simulink library "halout"  (R2021b)
settings: Solver=VariableStepAuto  StartTime=0.0  StopTime=10.0  RelTol=1e-3
undefined symbols (not defined in the file): C_TASK_5MS_S, FALSE, KHAL_CAN1FD1APS3E2E_flg, KHAL_CAN1FD1APS3TxReq_flg, KHAL_CAN1FD1VCU2E2E_flg, KHAL_CAN1FD1VCU2TxReq_flg, KHAL_CAN1FD1VCU3E2E_flg, KHAL_CAN1FD1VCU3TxReq_flg, KHAL_CAN1TxReq_flg, KHAL_CAN1VMCFCM1E2E_flg, KHAL_CAN1VMCFCM1TxReq_flg, KHAL_CAN2TxReq_flg, KHAL_CAN3FD3VCU1toNIDECTxReq_flg, KHAL_CAN3FD3VCU1TxReq_flg, KHAL_CAN3FD3VCU2E2E_flg, KHAL_CAN3FD3VCU2toNIDECE2E_flg, KHAL_CAN3FD3VCU2toNIDECTxReq_flg, KHAL_CAN3FD3VCU2TxReq_flg, KHAL_CAN3TxReq_flg, KHAL_CAN4FD4CE1000E2E_flg, KHAL_CAN4FD4CE1000TxReq_flg, KHAL_CAN4TxReq_flg, KHAL_CAN5TxReq_flg, KHAL_CAN6FD6APS3E2E_flg, KHAL_CAN6FD6APS3TxReq_flg, KHAL_CAN6FD6VCU2E2E_flg, KHAL_CAN6FD6VCU2TxReq_flg, KHAL_CAN6TxReq_flg, ONE_INT, TRUE, ZERO_INT
libraries: FVT_lib x549, simulink x244
(part 18 of 27)

== system halout/HAL_OUT/CAN2/FD2_CE100_0_0x117/FDCBCMHMIKey2FuncSta ==
  FDCBCMHMIKey2FuncSta : Inport
  Data Type Conversion : DataTypeConversion  OutDataTypeStr=uint8  RndMeth=Round
  CAN2_FDC_BCM_HMIKey2Func_Sta : Outport
  wires:
  Data Type Conversion/1 -> CAN2_FDC_BCM_HMIKey2Func_Sta/1
  FDCBCMHMIKey2FuncSta/1 -> Data Type Conversion/1

== system halout/HAL_OUT/CAN2/FD2_CE100_0_0x117/FDCBCMHMIKey3FuncSta ==
  FDCBCMHMIKey3FuncSta : Inport
  Data Type Conversion : DataTypeConversion  OutDataTypeStr=uint8  RndMeth=Round
  CAN2_FDC_BCM_HMIKey3Func_Sta : Outport
  wires:
  Data Type Conversion/1 -> CAN2_FDC_BCM_HMIKey3Func_Sta/1
  FDCBCMHMIKey3FuncSta/1 -> Data Type Conversion/1

== system halout/HAL_OUT/CAN2/FD2_CE100_0_0x117/FDCBCMHMIKey4FuncSta ==
  FDCBCMHMIKey4FuncSta : Inport
  Data Type Conversion : DataTypeConversion  OutDataTypeStr=uint8  RndMeth=Round
  CAN2_FDC_BCM_HMIKey4Func_Sta : Outport
  wires:
  Data Type Conversion/1 -> CAN2_FDC_BCM_HMIKey4Func_Sta/1
  FDCBCMHMIKey4FuncSta/1 -> Data Type Conversion/1

== system halout/HAL_OUT/CAN2/FD2_CE100_0_0x117/FDCBCMHMIKey5FuncSta ==
  FDCBCMHMIKey5FuncSta : Inport
  Data Type Conversion : DataTypeConversion  OutDataTypeStr=uint8  RndMeth=Round
  CAN2_FDC_BCM_HMIKey5Func_Sta : Outport
  wires:
  Data Type Conversion/1 -> CAN2_FDC_BCM_HMIKey5Func_Sta/1
  FDCBCMHMIKey5FuncSta/1 -> Data Type Conversion/1

== system halout/HAL_OUT/CAN2/FD2_CE100_0_0x117/FDCBCMHMIKey6FuncSta ==
  FDCBCMHMIKey6FuncSta : Inport
  Data Type Conversion : DataTypeConversion  OutDataTypeStr=uint8  RndMeth=Round
  CAN2_FDC_BCM_HMIKey6Func_Sta : Outport
  wires:
  Data Type Conversion/1 -> CAN2_FDC_BCM_HMIKey6Func_Sta/1
  FDCBCMHMIKey6FuncSta/1 -> Data Type Conversion/1

== system halout/HAL_OUT/CAN2/FD2_CE100_0_0x117/FDCBCMHMIKey7FuncSta ==
  FDCBCMHMIKey7FuncSta : Inport
  Data Type Conversion : DataTypeConversion  OutDataTypeStr=uint8  RndMeth=Round
  CAN2_FDC_BCM_HMIKey7Func_Sta : Outport
  wires:
  Data Type Conversion/1 -> CAN2_FDC_BCM_HMIKey7Func_Sta/1
  FDCBCMHMIKey7FuncSta/1 -> Data Type Conversion/1

== system halout/HAL_OUT/CAN2/FD2_CE100_0_0x117/FDCBCMHMIKey8FuncSta ==
  FDCBCMHMIKey8FuncSta : Inport
  Data Type Conversion : DataTypeConversion  OutDataTypeStr=uint8  RndMeth=Round
  CAN2_FDC_BCM_HMIKey8Func_Sta : Outport
  wires:
  Data Type Conversion/1 -> CAN2_FDC_BCM_HMIKey8Func_Sta/1
  FDCBCMHMIKey8FuncSta/1 -> Data Type Conversion/1

== system halout/HAL_OUT/CAN2/FD2_CE100_0_0x117/FDCRAPSErrWarnSta ==
  FDCRAPSErrWarnSta : Inport
  Data Type Conversion : DataTypeConversion  OutDataTypeStr=uint8  RndMeth=Round
  CAN2_FDC_RAPS_ErrWarn_Sta : Outport
  wires:
  Data Type Conversion/1 -> CAN2_FDC_RAPS_ErrWarn_Sta/1
  FDCRAPSErrWarnSta/1 -> Data Type Conversion/1

== system halout/HAL_OUT/CAN2/FD2_CE100_0_0x117/FDCTHCMCLEVentYSta ==
  FDCTHCMCLEVentYSta : Inport
  Data Type Conversion : DataTypeConversion  OutDataTypeStr=uint8  RndMeth=Round
  CAN2_FDC_THCM_CLEVentY_Sta : Outport
  wires:
  Data Type Conversion/1 -> CAN2_FDC_THCM_CLEVentY_Sta/1
  FDCTHCMCLEVentYSta/1 -> Data Type Conversion/1

== system halout/HAL_OUT/CAN2/FD2_CE100_0_0x117/FDCTHCMCLEVentZSta ==
  FDCTHCMCLEVentZSta : Inport
  Data Type Conversion : DataTypeConversion  OutDataTypeStr=uint8  RndMeth=Round
  CAN2_FDC_THCM_CLEVentZ_Sta : Outport
  wires:
  Data Type Conversion/1 -> CAN2_FDC_THCM_CLEVentZ_Sta/1
  FDCTHCMCLEVentZSta/1 -> Data Type Conversion/1

== system halout/HAL_OUT/CAN2/FD2_CE100_0_0x117/FDCTHCMCLVentSta ==
  FDCTHCMCLVentSta : Inport
  Data Type Conversion : DataTypeConversion  OutDataTypeStr=uint8  RndMeth=Round
  CAN2_FDC_THCM_CLVent_Sta : Outport
  wires:
  Data Type Conversion/1 -> CAN2_FDC_THCM_CLVent_Sta/1
  FDCTHCMCLVentSta/1 -> Data Type Conversion/1

== system halout/HAL_OUT/CAN2/FD2_CE100_0_0x117/FDCTHCMCREVentYSta ==
  FDCTHCMCREVentYSta : Inport
  Data Type Conversion : DataTypeConversion  OutDataTypeStr=uint8  RndMeth=Round
  CAN2_FDC_THCM_CREVentY_Sta : Outport
  wires:
  Data Type Conversion/1 -> CAN2_FDC_THCM_CREVentY_Sta/1
  FDCTHCMCREVentYSta/1 -> Data Type Conversion/1

== system halout/HAL_OUT/CAN2/FD2_CE100_0_0x117/FDCTHCMCREVentZSta ==
  FDCTHCMCREVentZSta : Inport
  Data Type Conversion : DataTypeConversion  OutDataTypeStr=uint8  RndMeth=Round
  CAN2_FDC_THCM_CREVentZ_Sta : Outport
  wires:
  Data Type Conversion/1 -> CAN2_FDC_THCM_CREVentZ_Sta/1
  FDCTHCMCREVentZSta/1 -> Data Type Conversion/1

== system halout/HAL_OUT/CAN2/FD2_CE100_0_0x117/FDCTHCMCRVentSta ==
  FDCTHCMCRVentSta : Inport
  Data Type Conversion : DataTypeConversion  OutDataTypeStr=uint8  RndMeth=Round
  CAN2_FDC_THCM_CRVent_Sta : Outport
  wires:
  Data Type Conversion/1 -> CAN2_FDC_THCM_CRVent_Sta/1
  FDCTHCMCRVentSta/1 -> Data Type Conversion/1

== system halout/HAL_OUT/CAN2/FD2_CE100_0_0x117/FDCTHCMDrEVentModeSta ==
  FDCTHCMDrEVentModeSta : Inport
  Data Type Conversion : DataTypeConversion  OutDataTypeStr=uint8  RndMeth=Round
  CAN2_FDC_THCM_DrEVentMode_Sta : Outport
  wires:
  Data Type Conversion/1 -> CAN2_FDC_THCM_DrEVentMode_Sta/1
  FDCTHCMDrEVentModeSta/1 -> Data Type Conversion/1

== system halout/HAL_OUT/CAN2/FD2_CE100_0_0x117/FDCTHCMDrEVentYSta ==
  FDCTHCMDrEVentYSta : Inport
  Data Type Conversion : DataTypeConversion  OutDataTypeStr=uint8  RndMeth=Round
  CAN2_FDC_THCM_DrEVentY_Sta : Outport
  wires:
  Data Type Conversion/1 -> CAN2_FDC_THCM_DrEVentY_Sta/1
  FDCTHCMDrEVentYSta/1 -> Data Type Conversion/1

== system halout/HAL_OUT/CAN2/FD2_CE100_0_0x117/FDCTHCMDrEVentZSta ==
  FDCTHCMDrEVentZSta : Inport
  Data Type Conversion : DataTypeConversion  OutDataTypeStr=uint8  RndMeth=Round
  CAN2_FDC_THCM_DrEVentZ_Sta : Outport
  wires:
  Data Type Conversion/1 -> CAN2_FDC_THCM_DrEVentZ_Sta/1
  FDCTHCMDrEVentZSta/1 -> Data Type Conversion/1

== system halout/HAL_OUT/CAN2/FD2_CE100_0_0x117/FDCTHCMDrVentSta ==
  FDCTHCMDrVentSta : Inport
  Data Type Conversion : DataTypeConversion  OutDataTypeStr=uint8  RndMeth=Round
  CAN2_FDC_THCM_DrVent_Sta : Outport
  wires:
  Data Type Conversion/1 -> CAN2_FDC_THCM_DrVent_Sta/1
  FDCTHCMDrVentSta/1 -> Data Type Conversion/1

== system halout/HAL_OUT/CAN2/FD2_CE100_0_0x117/FDCTHCMPreWPTCHeatSta ==
  FDCTHCMPreWPTCHeatSta : Inport
  Data Type Conversion : DataTypeConversion  OutDataTypeStr=uint8  RndMeth=Round
  CAN2_FDC_THCM_PreWPTCHeat_Sta : Outport
  wires:
  Data Type Conversion/1 -> CAN2_FDC_THCM_PreWPTCHeat_Sta/1
  FDCTHCMPreWPTCHeatSta/1 -> Data Type Conversion/1

== system halout/HAL_OUT/CAN2/FD2_CE100_0_0x117/FDCTHCMPsEVentModeSta ==
  FDCTHCMPsEVentModeSta : Inport
  Data Type Conversion : DataTypeConversion  OutDataTypeStr=uint8  RndMeth=Round
  CAN2_FDC_THCM_PsEVentMode_Sta : Outport
  wires:
  Data Type Conversion/1 -> CAN2_FDC_THCM_PsEVentMode_Sta/1
  FDCTHCMPsEVentModeSta/1 -> Data Type Conversion/1

== system halout/HAL_OUT/CAN2/FD2_CE100_0_0x117/FDCTHCMPsEVentYSta ==
  FDCTHCMPsEVentYSta : Inport
  Data Type Conversion : DataTypeConversion  OutDataTypeStr=uint8  RndMeth=Round
  CAN2_FDC_THCM_PsEVentY_Sta : Outport
  wires:
  Data Type Conversion/1 -> CAN2_FDC_THCM_PsEVentY_Sta/1
  FDCTHCMPsEVentYSta/1 -> Data Type Conversion/1

== system halout/HAL_OUT/CAN2/FD2_CE100_0_0x117/FDCTHCMPsEVentZSta ==
  FDCTHCMPsEVentZSta : Inport
  Data Type Conversion : DataTypeConversion  OutDataTypeStr=uint8  RndMeth=Round
  CAN2_FDC_THCM_PsEVentZ_Sta : Outport
  wires:
  Data Type Conversion/1 -> CAN2_FDC_THCM_PsEVentZ_Sta/1
  FDCTHCMPsEVentZSta/1 -> Data Type Conversion/1

== system halout/HAL_OUT/CAN2/FD2_CE100_0_0x117/FDCTHCMPsVentSta ==
  FDCTHCMPsVentSta : Inport
  Data Type Conversion : DataTypeConversion  OutDataTypeStr=uint8  RndMeth=Round
  CAN2_FDC_THCM_PsVent_Sta : Outport
  wires:
  Data Type Conversion/1 -> CAN2_FDC_THCM_PsVent_Sta/1
  FDCTHCMPsVentSta/1 -> Data Type Conversion/1

== system halout/HAL_OUT/CAN2/FD2_CE100_0_0x117/FDCV2LIVIV2LDischargCmd ==
  FDCV2LIVIV2LDischargCmd : Inport
  Data Type Conversion : DataTypeConversion  OutDataTypeStr=uint8  RndMeth=Round
  CAN2_FDC_V2L_IVIV2LDischarg_Cmd : Outport
  wires:
  Data Type Conversion/1 -> CAN2_FDC_V2L_IVIV2LDischarg_Cmd/1
  FDCV2LIVIV2LDischargCmd/1 -> Data Type Conversion/1

== system halout/HAL_OUT/CAN2/FD2_CE100_0_0x117/FDCVCULVChrgFreqSta ==
  FDCVCULVChrgFreqSta : Inport
  Data Type Conversion : DataTypeConversion  OutDataTypeStr=uint8  RndMeth=Round
  CAN2_FDC_VCU_LVChrgFreq_Sta : Outport
  wires:
  Data Type Conversion/1 -> CAN2_FDC_VCU_LVChrgFreq_Sta/1
  FDCVCULVChrgFreqSta/1 -> Data Type Conversion/1

== system halout/HAL_OUT/CAN2/FD2_CE100_0_0x117/FDCVCULVStaDropQuickSta ==
  FDCVCULVStaDropQuickSta : Inport
  Data Type Conversion : DataTypeConversion  OutDataTypeStr=uint8  RndMeth=Round
  CAN2_FDC_VCU_LVStaDropQuick_Sta : Outport
  wires:
  Data Type Conversion/1 -> CAN2_FDC_VCU_LVStaDropQuick_Sta/1
  FDCVCULVStaDropQuickSta/1 -> Data Type Conversion/1

== system halout/HAL_OUT/CAN2/FD2_CE100_0_0x117/FDCVCULVStaTooLowSta ==
  FDCVCULVStaTooLowSta : Inport
  Data Type Conversion : DataTypeConversion  OutDataTypeStr=uint8  RndMeth=Round
  CAN2_FDC_VCU_LVStaTooLow_Sta : Outport
  wires:
  Data Type Conversion/1 -> CAN2_FDC_VCU_LVStaTooLow_Sta/1
  FDCVCULVStaTooLowSta/1 -> Data Type Conversion/1

== system halout/HAL_OUT/CAN2/FD2_CE100_0_0x117/FDCVCUPwrSaveReqCmd ==
  FDCVCUPwrSaveReqCmd : Inport
  Data Type Conversion : DataTypeConversion  OutDataTypeStr=uint8  RndMeth=Round
  CAN2_FDC_VCU_PwrSaveReq_Cmd : Outport
  wires:
  Data Type Conversion/1 -> CAN2_FDC_VCU_PwrSaveReq_Cmd/1
  FDCVCUPwrSaveReqCmd/1 -> Data Type Conversion/1

== system halout/HAL_OUT/CAN2/FD2_CE100_0_0x117/FDCVCUTrailerDisOPDSta ==
  FDCVCUTrailerDisOPDSta : Inport
  Data Type Conversion : DataTypeConversion  OutDataTypeStr=uint8  RndMeth=Round
  CAN2_FDC_VCU_TrailerDisOPD_Sta : Outport
  wires:
  Data Type Conversion/1 -> CAN2_FDC_VCU_TrailerDisOPD_Sta/1
  FDCVCUTrailerDisOPDSta/1 -> Data Type Conversion/1

== system halout/HAL_OUT/CAN2/FD2_CE100_0_0x117/FDEBMErrSta ==
  FDEBMErrSta : Inport
  Data Type Conversion : DataTypeConversion  OutDataTypeStr=uint8  RndMeth=Round
  CAN2_FD_EBMErrSta : Outport
  wires:
  Data Type Conversion/1 -> CAN2_FD_EBMErrSta/1
  FDEBMErrSta/1 -> Data Type Conversion/1

== system halout/HAL_OUT/CAN2/FD2_CE100_0_0x117/FDEDriveSystem ==
  FDEDriveSystem : Inport
  Data Type Conversion : DataTypeConversion  OutDataTypeStr=uint8  RndMeth=Round
  CAN2_FD_EDrive_System : Outport
  wires:
  Data Type Conversion/1 -> CAN2_FD_EDrive_System/1
  FDEDriveSystem/1 -> Data Type Conversion/1

== system halout/HAL_OUT/CAN2/FD2_CE100_0_0x117/FDEPBError ==
  FDEPBError : Inport
  Data Type Conversion : DataTypeConversion  OutDataTypeStr=uint8  RndMeth=Round
  CAN2_FD_EPB_Error : Outport
  wires:
  Data Type Conversion/1 -> CAN2_FD_EPB_Error/1
  FDEPBError/1 -> Data Type Conversion/1

== system halout/HAL_OUT/CAN2/FD2_CE100_0_0x117/FDHVBatteryFault ==
  FDHVBatteryFault : Inport
  Data Type Conversion : DataTypeConversion  OutDataTypeStr=uint8  RndMeth=Round
  CAN2_FD_HV_Battery_Fault : Outport
  wires:
  Data Type Conversion/1 -> CAN2_FD_HV_Battery_Fault/1
  FDHVBatteryFault/1 -> Data Type Conversion/1

== system halout/HAL_OUT/CAN2/FD2_CE100_0_0x117/FDParkBrakeWarning ==
  FDParkBrakeWarning : Inport
  Data Type Conversion : DataTypeConversion  OutDataTypeStr=uint8  RndMeth=Round
  CAN2_FD_Park_Brake_Warning : Outport
  wires:
  Data Type Conversion/1 -> CAN2_FD_Park_Brake_Warning/1
  FDParkBrakeWarning/1 -> Data Type Conversion/1

== system halout/HAL_OUT/CAN2/FD2_CE100_0_0x117/FDPowerlimitation ==
  FDPowerlimitation : Inport
  Data Type Conversion : DataTypeConversion  OutDataTypeStr=uint8  RndMeth=Round
  CAN2_FD_Power_limitation : Outport
  wires:
  Data Type Conversion/1 -> CAN2_FD_Power_limitation/1
  FDPowerlimitation/1 -> Data Type Conversion/1

== system halout/HAL_OUT/CAN2/FD2_CE100_0_0x117/FDSteeringWarning ==
  FDSteeringWarning : Inport
  Data Type Conversion : DataTypeConversion  OutDataTypeStr=uint8  RndMeth=Round
  CAN2_FD_Steering_Warning : Outport
  wires:
  Data Type Conversion/1 -> CAN2_FD_Steering_Warning/1
  FDSteeringWarning/1 -> Data Type Conversion/1

== system halout/HAL_OUT/CAN2/FD2_CE100_0_0x117/FDTCSIndicator ==
  FDTCSIndicator : Inport
  Data Type Conversion : DataTypeConversion  OutDataTypeStr=uint8  RndMeth=Round
  CAN2_FD_TCS_Indicator : Outport
  wires:
  Data Type Conversion/1 -> CAN2_FD_TCS_Indicator/1
  FDTCSIndicator/1 -> Data Type Conversion/1

== system halout/HAL_OUT/CAN2/FD2_CE100_0_0x117/FDTelltaleFail ==
  FDTelltaleFail : Inport
  Data Type Conversion : DataTypeConversion  OutDataTypeStr=uint8  RndMeth=Round
  CAN2_FD_Telltale_Fail : Outport
  wires:
  Data Type Conversion/1 -> CAN2_FD_Telltale_Fail/1
  FDTelltaleFail/1 -> Data Type Conversion/1

== system halout/HAL_OUT/CAN2/FD2_CE100_0_0x117/FalseNPreventSta ==
  FalseNPreventSta : Inport
  Data Type Conversion : DataTypeConversion  OutDataTypeStr=uint8  RndMeth=Round
  CAN2_FalseNPrevent_Sta : Outport
  wires:
  Data Type Conversion/1 -> CAN2_FalseNPrevent_Sta/1
  FalseNPreventSta/1 -> Data Type Conversion/1

== system halout/HAL_OUT/CAN2/FD2_CE100_0_0x117/FeatSetSpdFinalraw32 ==
  FeatSetSpdFinalraw32 : Inport
  Data Type Conversion : DataTypeConversion  OutDataTypeStr=uint8  RndMeth=Round
  CAN2_FeatSetSpdFinal_raw32 : Outport
  wires:
  Data Type Conversion/1 -> CAN2_FeatSetSpdFinal_raw32/1
  FeatSetSpdFinalraw32/1 -> Data Type Conversion/1

== system halout/HAL_OUT/CAN2/FD2_CE100_0_0x117/FollowMe ==
  FollowMe : Inport
  Data Type Conversion : DataTypeConversion  OutDataTypeStr=uint8  RndMeth=Round
  CAN2_FollowMe : Outport
  wires:
  Data Type Conversion/1 -> CAN2_FollowMe/1
  FollowMe/1 -> Data Type Conversion/1

== system halout/HAL_OUT/CAN2/FD2_CE100_0_0x117/FrFogLamp ==
  FrFogLamp : Inport
  Data Type Conversion : DataTypeConversion  OutDataTypeStr=uint8  RndMeth=Round
  CAN2_Fr_FogLamp : Outport
  wires:
  Data Type Conversion/1 -> CAN2_Fr_FogLamp/1
  FrFogLamp/1 -> Data Type Conversion/1

== system halout/HAL_OUT/CAN2/FD2_CE100_0_0x117/HBeam ==
  HBeam : Inport
  Data Type Conversion : DataTypeConversion  OutDataTypeStr=uint8  RndMeth=Round
  CAN2_H_Beam : Outport
  wires:
  Data Type Conversion/1 -> CAN2_H_Beam/1
  HBeam/1 -> Data Type Conversion/1

== system halout/HAL_OUT/CAN2/FD2_CE100_0_0x117/HVRlyOpFail ==
  HVRlyOpFail : Inport
  Data Type Conversion : DataTypeConversion  OutDataTypeStr=uint8  RndMeth=Round
  CAN2_HVRlyOpFail : Outport
  wires:
  Data Type Conversion/1 -> CAN2_HVRlyOpFail/1
  HVRlyOpFail/1 -> Data Type Conversion/1

== system halout/HAL_OUT/CAN2/FD2_CE100_0_0x117/HVSysErrIsolationErr ==
  HVSysErrIsolationErr : Inport
  Data Type Conversion : DataTypeConversion  OutDataTypeStr=uint8  RndMeth=Round
  CAN2_HVSysErr_IsolationErr : Outport
  wires:
  Data Type Conversion/1 -> CAN2_HVSysErr_IsolationErr/1
  HVSysErrIsolationErr/1 -> Data Type Conversion/1

== system halout/HAL_OUT/CAN2/FD2_CE100_0_0x117/HVSysErrPackErr ==
  HVSysErrPackErr : Inport
  Data Type Conversion : DataTypeConversion  OutDataTypeStr=uint8  RndMeth=Round
  CAN2_HVSysErr_PackErr : Outport
  wires:
  Data Type Conversion/1 -> CAN2_HVSysErr_PackErr/1
  HVSysErrPackErr/1 -> Data Type Conversion/1

== system halout/HAL_OUT/CAN2/FD2_CE100_0_0x117/HVSysErrRelayErr ==
  HVSysErrRelayErr : Inport
  Data Type Conversion : DataTypeConversion  OutDataTypeStr=uint8  RndMeth=Round
  CAN2_HVSysErr_RelayErr : Outport
  wires:
  Data Type Conversion/1 -> CAN2_HVSysErr_RelayErr/1
  HVSysErrRelayErr/1 -> Data Type Conversion/1

== system halout/HAL_OUT/CAN2/FD2_CE100_0_0x117/HazardSW ==
  HazardSW : Inport
  Data Type Conversion : DataTypeConversion  OutDataTypeStr=uint8  RndMeth=Round
  CAN2_HazardSW : Outport
  wires:
  Data Type Conversion/1 -> CAN2_HazardSW/1
  HazardSW/1 -> Data Type Conversion/1

== system halout/HAL_OUT/CAN2/FD2_CE100_0_0x117/HoodSW ==
  HoodSW : Inport
  Data Type Conversion : DataTypeConversion  OutDataTypeStr=uint8  RndMeth=Round
  CAN2_HoodSW : Outport
  wires:
  Data Type Conversion/1 -> CAN2_HoodSW/1
  HoodSW/1 -> Data Type Conversion/1

== system halout/HAL_OUT/CAN2/FD2_CE100_0_0x117/LBSD ==
  LBSD : Inport
  Data Type Conversion : DataTypeConversion  OutDataTypeStr=uint8  RndMeth=Round
  CAN2_LBSD : Outport
  wires:
  Data Type Conversion/1 -> CAN2_LBSD/1
  LBSD/1 -> Data Type Conversion/1

== system halout/HAL_OUT/CAN2/FD2_CE100_0_0x117/LBeam ==
  LBeam : Inport
  Data Type Conversion : DataTypeConversion  OutDataTypeStr=uint8  RndMeth=Round
  CAN2_L_Beam : Outport
  wires:
  Data Type Conversion/1 -> CAN2_L_Beam/1
  LBeam/1 -> Data Type Conversion/1

== system halout/HAL_OUT/CAN2/FD2_CE100_0_0x117/LDRL ==
  LDRL : Inport
  Data Type Conversion : DataTypeConversion  OutDataTypeStr=uint8  RndMeth=Round
  CAN2_LDRL : Outport
  wires:
  Data Type Conversion/1 -> CAN2_LDRL/1
  LDRL/1 -> Data Type Conversion/1

== system halout/HAL_OUT/CAN2/FD2_CE100_0_0x117/LTurnLP ==
  LTurnLP : Inport
  Data Type Conversion : DataTypeConversion  OutDataTypeStr=uint8  RndMeth=Round
  CAN2_LTurnLP : Outport
  wires:
  Data Type Conversion/1 -> CAN2_LTurnLP/1
  LTurnLP/1 -> Data Type Conversion/1

== system halout/HAL_OUT/CAN2/FD2_CE100_0_0x117/LVChrgFuncStaChk ==
  LVChrgFuncStaChk : Inport
  Data Type Conversion : DataTypeConversion  OutDataTypeStr=uint8  RndMeth=Round
  CAN2_LVChrgFuncStaChk : Outport
  wires:
  Data Type Conversion/1 -> CAN2_LVChrgFuncStaChk/1
  LVChrgFuncStaChk/1 -> Data Type Conversion/1

== system halout/HAL_OUT/CAN2/FD2_CE100_0_0x117/LVSilentChrgReq ==
  LVSilentChrgReq : Inport
  Data Type Conversion : DataTypeConversion  OutDataTypeStr=uint8  RndMeth=Round
  CAN2_LVSilentChrgReq : Outport
  wires:
  Data Type Conversion/1 -> CAN2_LVSilentChrgReq/1
  LVSilentChrgReq/1 -> Data Type Conversion/1

== system halout/HAL_OUT/CAN2/FD2_CE100_0_0x117/LVSilentChrgSta ==
  LVSilentChrgSta : Inport
  Data Type Conversion : DataTypeConversion  OutDataTypeStr=uint8  RndMeth=Round
  CAN2_LVSilentChrgSta : Outport
  wires:
  Data Type Conversion/1 -> CAN2_LVSilentChrgSta/1
  LVSilentChrgSta/1 -> Data Type Conversion/1

== system halout/HAL_OUT/CAN2/FD2_CE100_0_0x117/LVSysErrPwrOutpErr ==
  LVSysErrPwrOutpErr : Inport
  Data Type Conversion : DataTypeConversion  OutDataTypeStr=uint8  RndMeth=Round
  CAN2_LVSysErr_PwrOutpErr : Outport
  wires:
  Data Type Conversion/1 -> CAN2_LVSysErr_PwrOutpErr/1
  LVSysErrPwrOutpErr/1 -> Data Type Conversion/1

== system halout/HAL_OUT/CAN2/FD2_CE100_0_0x117/LimphomeAct ==
  LimphomeAct : Inport
  Data Type Conversion : DataTypeConversion  OutDataTypeStr=uint8  RndMeth=Round
  CAN2_LimphomeAct : Outport
  wires:
  Data Type Conversion/1 -> CAN2_LimphomeAct/1
  LimphomeAct/1 -> Data Type Conversion/1

== system halout/HAL_OUT/CAN2/FD2_CE100_0_0x117/LockSetting ==
  LockSetting : Inport
  Data Type Conversion : DataTypeConversion  OutDataTypeStr=uint8  RndMeth=Round
  CAN2_LockSetting : Outport
  wires:
  Data Type Conversion/1 -> CAN2_LockSetting/1
  LockSetting/1 -> Data Type Conversion/1

== system halout/HAL_OUT/CAN2/FD2_CE100_0_0x117/MCUActDisFail ==
  MCUActDisFail : Inport
  Data Type Conversion : DataTypeConversion  OutDataTypeStr=uint8  RndMeth=Round
  CAN2_MCUActDisFail : Outport
  wires:
  Data Type Conversion/1 -> CAN2_MCUActDisFail/1
  MCUActDisFail/1 -> Data Type Conversion/1

== system halout/HAL_OUT/CAN2/FD2_CE100_0_0x117/MSACrlSta ==
  MSACrlSta : Inport
  Data Type Conversion : DataTypeConversion  OutDataTypeStr=uint8  RndMeth=Round
  CAN2_MSA_Crl_Sta : Outport
  wires:
  Data Type Conversion/1 -> CAN2_MSA_Crl_Sta/1
  MSACrlSta/1 -> Data Type Conversion/1

== system halout/HAL_OUT/CAN2/FD2_CE100_0_0x117/MeterIndSpeedraw32 ==
  MeterIndSpeedraw32 : Inport
  Data Type Conversion : DataTypeConversion  OutDataTypeStr=uint8  RndMeth=Round
  CAN2_MeterIndSpeed_raw32 : Outport
  wires:
  Data Type Conversion/1 -> CAN2_MeterIndSpeed_raw32/1
  MeterIndSpeedraw32/1 -> Data Type Conversion/1

== system halout/HAL_OUT/CAN2/FD2_CE100_0_0x117/PASStaFSys ==
  PASStaFSys : Inport
  Data Type Conversion : DataTypeConversion  OutDataTypeStr=uint8  RndMeth=Round
  CAN2_PAS_Sta_F_Sys : Outport
  wires:
  Data Type Conversion/1 -> CAN2_PAS_Sta_F_Sys/1
  PASStaFSys/1 -> Data Type Conversion/1

== system halout/HAL_OUT/CAN2/FD2_CE100_0_0x117/PosLamp ==
  PosLamp : Inport
  Data Type Conversion : DataTypeConversion  OutDataTypeStr=uint8  RndMeth=Round
  CAN2_PosLamp : Outport
  wires:
  Data Type Conversion/1 -> CAN2_PosLamp/1
  PosLamp/1 -> Data Type Conversion/1

== system halout/HAL_OUT/CAN2/FD2_CE100_0_0x117/PsDoorSW ==
  PsDoorSW : Inport
  Data Type Conversion : DataTypeConversion  OutDataTypeStr=uint8  RndMeth=Round
  CAN2_PsDoorSW : Outport
  wires:
  Data Type Conversion/1 -> CAN2_PsDoorSW/1
  PsDoorSW/1 -> Data Type Conversion/1

== system halout/HAL_OUT/CAN2/FD2_CE100_0_0x117/PwrSta ==
  PwrSta : Inport
  Data Type Conversion : DataTypeConversion  OutDataTypeStr=uint8  RndMeth=Round
  CAN2_PwrSta : Outport
  wires:
  Data Type Conversion/1 -> CAN2_PwrSta/1
  PwrSta/1 -> Data Type Conversion/1

== system halout/HAL_OUT/CAN2/FD2_CE100_0_0x117/PwrStaErr ==
  PwrStaErr : Inport
  Data Type Conversion : DataTypeConversion  OutDataTypeStr=uint8  RndMeth=Round
  CAN2_PwrStaErr : Outport
  wires:
  Data Type Conversion/1 -> CAN2_PwrStaErr/1
  PwrStaErr/1 -> Data Type Conversion/1

== system halout/HAL_OUT/CAN2/FD2_CE100_0_0x117/PwrStaONTOIVIPopReq ==
  PwrStaONTOIVIPopReq : Inport
  Data Type Conversion : DataTypeConversion  OutDataTypeStr=uint8  RndMeth=Round
  CAN2_PwrStaONTOIVIPopReq : Outport
  wires:
  Data Type Conversion/1 -> CAN2_PwrStaONTOIVIPopReq/1
  PwrStaONTOIVIPopReq/1 -> Data Type Conversion/1

== system halout/HAL_OUT/CAN2/FD2_CE100_0_0x117/PwrStaONTOIVIPopT ==
  PwrStaONTOIVIPopT : Inport
  Data Type Conversion : DataTypeConversion  OutDataTypeStr=uint16  RndMeth=Round
  CAN2_PwrStaONTOIVIPopT : Outport
  wires:
  Data Type Conversion/1 -> CAN2_PwrStaONTOIVIPopT/1
  PwrStaONTOIVIPopT/1 -> Data Type Conversion/1

== system halout/HAL_OUT/CAN2/FD2_CE100_0_0x117/RBSD ==
  RBSD : Inport
  Data Type Conversion : DataTypeConversion  OutDataTypeStr=uint8  RndMeth=Round
  CAN2_RBSD : Outport
  wires:
  Data Type Conversion/1 -> CAN2_RBSD/1
  RBSD/1 -> Data Type Conversion/1

== system halout/HAL_OUT/CAN2/FD2_CE100_0_0x117/RDRL ==
  RDRL : Inport
  Data Type Conversion : DataTypeConversion  OutDataTypeStr=uint8  RndMeth=Round
  CAN2_RDRL : Outport
  wires:
  Data Type Conversion/1 -> CAN2_RDRL/1
  RDRL/1 -> Data Type Conversion/1

== system halout/HAL_OUT/CAN2/FD2_CE100_0_0x117/RLDoorSW ==
  RLDoorSW : Inport
  Data Type Conversion : DataTypeConversion  OutDataTypeStr=uint8  RndMeth=Round
  CAN2_RLDoorSW : Outport
  wires:
  Data Type Conversion/1 -> CAN2_RLDoorSW/1
  RLDoorSW/1 -> Data Type Conversion/1

== system halout/HAL_OUT/CAN2/FD2_CE100_0_0x117/RRDoorSW ==
  RRDoorSW : Inport
  Data Type Conversion : DataTypeConversion  OutDataTypeStr=uint8  RndMeth=Round
  CAN2_RRDoorSW : Outport
  wires:
  Data Type Conversion/1 -> CAN2_RRDoorSW/1
  RRDoorSW/1 -> Data Type Conversion/1

== system halout/HAL_OUT/CAN2/FD2_CE100_0_0x117/RTurnLP ==
  RTurnLP : Inport
  Data Type Conversion : DataTypeConversion  OutDataTypeStr=uint8  RndMeth=Round
  CAN2_RTurnLP : Outport
  wires:
  Data Type Conversion/1 -> CAN2_RTurnLP/1
  RTurnLP/1 -> Data Type Conversion/1

== system halout/HAL_OUT/CAN2/FD2_CE100_0_0x117/ReqInternalV2LStatusLamp ==
  ReqInternalV2LStatusLamp : Inport
  Data Type Conversion : DataTypeConversion  OutDataTypeStr=uint8  RndMeth=Round
  CAN2_Req_Internal_V2L_Status_Lamp : Outport
  wires:
  Data Type Conversion/1 -> CAN2_Req_Internal_V2L_Status_Lamp/1
  ReqInternalV2LStatusLamp/1 -> Data Type Conversion/1

== system halout/HAL_OUT/CAN2/FD2_CE100_0_0x117/ReqV2LIVIPopup ==
  ReqV2LIVIPopup : Inport
  Data Type Conversion : DataTypeConversion  OutDataTypeStr=uint8  RndMeth=Round
  CAN2_Req_V2L_IVI_Popup : Outport
  wires:
  Data Type Conversion/1 -> CAN2_Req_V2L_IVI_Popup/1
  ReqV2LIVIPopup/1 -> Data Type Conversion/1

== system halout/HAL_OUT/CAN2/FD2_CE100_0_0x117/ReqV2LSwOn ==
  ReqV2LSwOn : Inport
  Data Type Conversion : DataTypeConversion  OutDataTypeStr=uint8  RndMeth=Round
  CAN2_Req_V2LSwOn : Outport
  wires:
  Data Type Conversion/1 -> CAN2_Req_V2LSwOn/1
  ReqV2LSwOn/1 -> Data Type Conversion/1

== system halout/HAL_OUT/CAN2/FD2_CE100_0_0x117/ReverseLamp ==
  ReverseLamp : Inport
  Data Type Conversion : DataTypeConversion  OutDataTypeStr=uint8  RndMeth=Round
  CAN2_ReverseLamp : Outport
  wires:
  Data Type Conversion/1 -> CAN2_ReverseLamp/1
  ReverseLamp/1 -> Data Type Conversion/1

== system halout/HAL_OUT/CAN2/FD2_CE100_0_0x117/RrDefog ==
  RrDefog : Inport
  Data Type Conversion : DataTypeConversion  OutDataTypeStr=uint8  RndMeth=Round
  CAN2_Rr_Defog : Outport
  wires:
  Data Type Conversion/1 -> CAN2_Rr_Defog/1
  RrDefog/1 -> Data Type Conversion/1

== system halout/HAL_OUT/CAN2/FD2_CE100_0_0x117/RrFogLamp ==
  RrFogLamp : Inport
  Data Type Conversion : DataTypeConversion  OutDataTypeStr=uint8  RndMeth=Round
  CAN2_Rr_FogLamp : Outport
  wires:
  Data Type Conversion/1 -> CAN2_Rr_FogLamp/1
  RrFogLamp/1 -> Data Type Conversion/1

== system halout/HAL_OUT/CAN2/FD2_CE100_0_0x117/ShiftGearPosn ==
  ShiftGearPosn : Inport
  Data Type Conversion : DataTypeConversion  OutDataTypeStr=uint8  RndMeth=Round
  CAN2_ShiftGearPosn : Outport
  wires:
  Data Type Conversion/1 -> CAN2_ShiftGearPosn/1
  ShiftGearPosn/1 -> Data Type Conversion/1

== system halout/HAL_OUT/CAN2/FD2_CE100_0_0x117/SysAllowReadySta ==
  SysAllowReadySta : Inport
  Data Type Conversion : DataTypeConversion  OutDataTypeStr=uint8  RndMeth=Round
  CAN2_SysAllowReadySta : Outport
  wires:
  Data Type Conversion/1 -> CAN2_SysAllowReadySta/1
  SysAllowReadySta/1 -> Data Type Conversion/1

== system halout/HAL_OUT/CAN2/FD2_CE100_0_0x117/SysPwrSta ==
  SysPwrSta : Inport
  Data Type Conversion : DataTypeConversion  OutDataTypeStr=uint8  RndMeth=Round
  CAN2_SysPwrSta : Outport
  wires:
  Data Type Conversion/1 -> CAN2_SysPwrSta/1
  SysPwrSta/1 -> Data Type Conversion/1

== system halout/HAL_OUT/CAN2/FD2_CE100_0_0x117/TailgateSW ==
  TailgateSW : Inport
  Data Type Conversion : DataTypeConversion  OutDataTypeStr=uint8  RndMeth=Round
  CAN2_Tailgate_SW : Outport
  wires:
  Data Type Conversion/1 -> CAN2_Tailgate_SW/1
  TailgateSW/1 -> Data Type Conversion/1

== system halout/HAL_OUT/CAN2/FD2_CE100_0_0x117/VCUBrkSWSta ==
  VCUBrkSWSta : Inport
  Data Type Conversion : DataTypeConversion  OutDataTypeStr=uint8  RndMeth=Round
  CAN2_VCUBrkSWSta : Outport
  wires:
  Data Type Conversion/1 -> CAN2_VCUBrkSWSta/1
  VCUBrkSWSta/1 -> Data Type Conversion/1

== system halout/HAL_OUT/CAN2/FD2_CE100_0_0x117/VCUFLDoorSta ==
  VCUFLDoorSta : Inport
  Data Type Conversion : DataTypeConversion  OutDataTypeStr=uint8  RndMeth=Round
  CAN2_VCUFLDoorSta : Outport
  wires:
  Data Type Conversion/1 -> CAN2_VCUFLDoorSta/1
  VCUFLDoorSta/1 -> Data Type Conversion/1

== system halout/HAL_OUT/CAN2/FD2_CE100_0_0x117/VCUFRDoorSta ==
  VCUFRDoorSta : Inport
  Data Type Conversion : DataTypeConversion  OutDataTypeStr=uint8  RndMeth=Round
  CAN2_VCUFRDoorSta : Outport
  wires:
  Data Type Conversion/1 -> CAN2_VCUFRDoorSta/1
  VCUFRDoorSta/1 -> Data Type Conversion/1

== system halout/HAL_OUT/CAN2/FD2_CE100_0_0x117/VCUHoodSWSta ==
  VCUHoodSWSta : Inport
  Data Type Conversion : DataTypeConversion  OutDataTypeStr=uint8  RndMeth=Round
  CAN2_VCUHoodSWSta : Outport
  wires:
  Data Type Conversion/1 -> CAN2_VCUHoodSWSta/1
  VCUHoodSWSta/1 -> Data Type Conversion/1

== system halout/HAL_OUT/CAN2/FD2_CE100_0_0x117/VCUOPDHold ==
  VCUOPDHold : Inport
  Data Type Conversion : DataTypeConversion  OutDataTypeStr=uint8  RndMeth=Round
  CAN2_VCU_OPDHold : Outport
  wires:
  Data Type Conversion/1 -> CAN2_VCU_OPDHold/1
  VCUOPDHold/1 -> Data Type Conversion/1

== system halout/HAL_OUT/CAN2/FD2_CE100_0_0x117/VCURLDoorSta ==
  VCURLDoorSta : Inport
  Data Type Conversion : DataTypeConversion  OutDataTypeStr=uint8  RndMeth=Round
  CAN2_VCURLDoorSta : Outport
  wires:
  Data Type Conversion/1 -> CAN2_VCURLDoorSta/1
  VCURLDoorSta/1 -> Data Type Conversion/1

== system halout/HAL_OUT/CAN2/FD2_CE100_0_0x117/VCURRDoorSta ==
  VCURRDoorSta : Inport
  Data Type Conversion : DataTypeConversion  OutDataTypeStr=uint8  RndMeth=Round
  CAN2_VCURRDoorSta : Outport
  wires:
  Data Type Conversion/1 -> CAN2_VCURRDoorSta/1
  VCURRDoorSta/1 -> Data Type Conversion/1

== system halout/HAL_OUT/CAN2/FD2_CE100_0_0x117/VCUTailgateSWSta ==
  VCUTailgateSWSta : Inport
  Data Type Conversion : DataTypeConversion  OutDataTypeStr=uint8  RndMeth=Round
  CAN2_VCUTailgateSWSta : Outport
  wires:
  Data Type Conversion/1 -> CAN2_VCUTailgateSWSta/1
  VCUTailgateSWSta/1 -> Data Type Conversion/1

== system halout/HAL_OUT/CAN2/FD2_CE100_0_0x117/VehMalfunLevel ==
  VehMalfunLevel : Inport
  Data Type Conversion : DataTypeConversion  OutDataTypeStr=uint8  RndMeth=Round
  CAN2_VehMalfunLevel : Outport
  wires:
  Data Type Conversion/1 -> CAN2_VehMalfunLevel/1
  VehMalfunLevel/1 -> Data Type Conversion/1

== system halout/HAL_OUT/CAN2/FD2_CE100_0_0x117/XWDMode ==
  XWDMode : Inport
  Data Type Conversion : DataTypeConversion  OutDataTypeStr=uint8  RndMeth=Round
  CAN2_XWDMode : Outport
  wires:
  Data Type Conversion/1 -> CAN2_XWDMode/1
  XWDMode/1 -> Data Type Conversion/1

== system halout/HAL_OUT/CAN2/FD2_CE100_0_0x117/sigAirIntenZon1St ==
  sigAirIntenZon1St : Inport
  Data Type Conversion : DataTypeConversion  OutDataTypeStr=uint8  RndMeth=Round
  CAN2_sigAirIntenZon1St : Outport
  wires:
  Data Type Conversion/1 -> CAN2_sigAirIntenZon1St/1
  sigAirIntenZon1St/1 -> Data Type Conversion/1

== system halout/HAL_OUT/CAN2/FD2_CE100_0_0x117/sigAirIntenZon3St ==
  sigAirIntenZon3St : Inport
  Data Type Conversion : DataTypeConversion  OutDataTypeStr=uint8  RndMeth=Round
  CAN2_sigAirIntenZon3St : Outport
  wires:
  Data Type Conversion/1 -> CAN2_sigAirIntenZon3St/1
  sigAirIntenZon3St/1 -> Data Type Conversion/1

== system halout/HAL_OUT/CAN2/FD2_CE100_0_0x117/sigAmbAirT ==
  sigAmbAirT : Inport
  Data Type Conversion : DataTypeConversion  OutDataTypeStr=uint8  RndMeth=Round
  convert_out : FVT_lib/hal/convert_out  gain=0.5  offset=-40
  CAN2_sigAmbAirT : Outport
  wires:
  Data Type Conversion/1 -> CAN2_sigAmbAirT/1
  convert_out/1 -> Data Type Conversion/1
  sigAmbAirT/1 -> convert_out/1

== system halout/HAL_OUT/CAN2/FD2_CE100_0_0x117/sigCbnAirT ==
  sigCbnAirT : Inport
  Data Type Conversion : DataTypeConversion  OutDataTypeStr=uint8  RndMeth=Round
  convert_out : FVT_lib/hal/convert_out  gain=0.5  offset=-40
  CAN2_sigCbnAirT : Outport
  wires:
  Data Type Conversion/1 -> CAN2_sigCbnAirT/1
  convert_out/1 -> Data Type Conversion/1
  sigCbnAirT/1 -> convert_out/1

== system halout/HAL_OUT/CAN2/FD2_CE100_0_0x117/sigDfrstSt ==
  sigDfrstSt : Inport
  Data Type Conversion : DataTypeConversion  OutDataTypeStr=uint8  RndMeth=Round
  CAN2_sigDfrstSt : Outport
  wires:
  Data Type Conversion/1 -> CAN2_sigDfrstSt/1
  sigDfrstSt/1 -> Data Type Conversion/1

== system halout/HAL_OUT/CAN2/FD2_CE100_0_0x117/sigHvacSt ==
  sigHvacSt : Inport
  Data Type Conversion : DataTypeConversion  OutDataTypeStr=uint8  RndMeth=Round
  CAN2_sigHvacSt : Outport
  wires:
  Data Type Conversion/1 -> CAN2_sigHvacSt/1
  sigHvacSt/1 -> Data Type Conversion/1

== system halout/HAL_OUT/CAN2/FD2_CE100_0_0x117/sigRecircSt ==
  sigRecircSt : Inport
  Data Type Conversion : DataTypeConversion  OutDataTypeStr=uint8  RndMeth=Round
  CAN2_sigRecircSt : Outport
  wires:
  Data Type Conversion/1 -> CAN2_sigRecircSt/1
  sigRecircSt/1 -> Data Type Conversion/1

== system halout/HAL_OUT/CAN2/FD2_CE100_0_0x117/sigSetTempZon1St ==
  sigSetTempZon1St : Inport
  Data Type Conversion : DataTypeConversion  OutDataTypeStr=uint8  RndMeth=Round
  convert_out : FVT_lib/hal/convert_out  gain=0.5  offset=17
  CAN2_sigSetTempZon1St : Outport
  wires:
  Data Type Conversion/1 -> CAN2_sigSetTempZon1St/1
  convert_out/1 -> Data Type Conversion/1
  sigSetTempZon1St/1 -> convert_out/1

== system halout/HAL_OUT/CAN2/FD2_CE100_0_0x117/sigSetTempZon2St ==
  sigSetTempZon2St : Inport
  Data Type Conversion : DataTypeConversion  OutDataTypeStr=uint8  RndMeth=Round
  convert_out : FVT_lib/hal/convert_out  gain=0.5  offset=17
  CAN2_sigSetTempZon2St : Outport
  wires:
  Data Type Conversion/1 -> CAN2_sigSetTempZon2St/1
  convert_out/1 -> Data Type Conversion/1
  sigSetTempZon2St/1 -> convert_out/1

== system halout/HAL_OUT/CAN2/FD2_CE100_0_0x117/sigSetTempZon3St ==
  sigSetTempZon3St : Inport
  Data Type Conversion : DataTypeConversion  OutDataTypeStr=uint8  RndMeth=Round
  convert_out : FVT_lib/hal/convert_out  gain=0.5  offset=17
  CAN2_sigSetTempZon3St : Outport
  wires:
  Data Type Conversion/1 -> CAN2_sigSetTempZon3St/1
  convert_out/1 -> Data Type Conversion/1
  sigSetTempZon3St/1 -> convert_out/1

== system halout/HAL_OUT/CAN2/FD2_CE100_0_0x117/sigWindDirZon1St ==
  sigWindDirZon1St : Inport
  Data Type Conversion : DataTypeConversion  OutDataTypeStr=uint8  RndMeth=Round
  CAN2_sigWindDirZon1St : Outport
  wires:
  Data Type Conversion/1 -> CAN2_sigWindDirZon1St/1
  sigWindDirZon1St/1 -> Data Type Conversion/1

== system halout/HAL_OUT/CAN2/FD2_CE100_0_0x117/sigWindDirZon3St ==
  sigWindDirZon3St : Inport
  Data Type Conversion : DataTypeConversion  OutDataTypeStr=uint8  RndMeth=Round
  CAN2_sigWindDirZon3St : Outport
  wires:
  Data Type Conversion/1 -> CAN2_sigWindDirZon3St/1
  sigWindDirZon3St/1 -> Data Type Conversion/1

== system halout/HAL_OUT/CAN2/FD2_CE200_1_0x435/AutoLTips ==
  AutoLTips : Inport
  Data Type Conversion : DataTypeConversion  OutDataTypeStr=uint8  RndMeth=Round
  CAN2_AutoLTips : Outport
  wires:
  Data Type Conversion/1 -> CAN2_AutoLTips/1
  AutoLTips/1 -> Data Type Conversion/1

== system halout/HAL_OUT/CAN2/FD2_CE200_1_0x435/CWheelTips ==
  CWheelTips : Inport
  Data Type Conversion : DataTypeConversion  OutDataTypeStr=uint8  RndMeth=Round
  CAN2_CWheelTips : Outport
  wires:
  Data Type Conversion/1 -> CAN2_CWheelTips/1
  CWheelTips/1 -> Data Type Conversion/1

== system halout/HAL_OUT/CAN2/FD2_CE200_1_0x435/FDCBCMAcc1StaSta ==
  FDCBCMAcc1StaSta : Inport
  Data Type Conversion : DataTypeConversion  OutDataTypeStr=uint8  RndMeth=Round
  CAN2_FDC_BCM_Acc1Sta_Sta : Outport
  wires:
  Data Type Conversion/1 -> CAN2_FDC_BCM_Acc1Sta_Sta/1
  FDCBCMAcc1StaSta/1 -> Data Type Conversion/1

== system halout/HAL_OUT/CAN2/FD2_CE200_1_0x435/FDCBCMAcc2StaSta ==
  FDCBCMAcc2StaSta : Inport
  Data Type Conversion : DataTypeConversion  OutDataTypeStr=uint8  RndMeth=Round
  CAN2_FDC_BCM_Acc2Sta_Sta : Outport
  wires:
  Data Type Conversion/1 -> CAN2_FDC_BCM_Acc2Sta_Sta/1
  FDCBCMAcc2StaSta/1 -> Data Type Conversion/1

== system halout/HAL_OUT/CAN2/FD2_CE200_1_0x435/FDCBCMAcc3StaSta ==
  FDCBCMAcc3StaSta : Inport
  Data Type Conversion : DataTypeConversion  OutDataTypeStr=uint8  RndMeth=Round
  CAN2_FDC_BCM_Acc3Sta_Sta : Outport
  wires:
  Data Type Conversion/1 -> CAN2_FDC_BCM_Acc3Sta_Sta/1
  FDCBCMAcc3StaSta/1 -> Data Type Conversion/1

== system halout/HAL_OUT/CAN2/FD2_CE200_1_0x435/FDCBCMAcc4StaSta ==
  FDCBCMAcc4StaSta : Inport
  Data Type Conversion : DataTypeConversion  OutDataTypeStr=uint8  RndMeth=Round
  CAN2_FDC_BCM_Acc4Sta_Sta : Outport
  wires:
  Data Type Conversion/1 -> CAN2_FDC_BCM_Acc4Sta_Sta/1
  FDCBCMAcc4StaSta/1 -> Data Type Conversion/1

== system halout/HAL_OUT/CAN2/FD2_CE200_1_0x435/FDCBCMAcc5StaSta ==
  FDCBCMAcc5StaSta : Inport
  Data Type Conversion : DataTypeConversion  OutDataTypeStr=uint8  RndMeth=Round
  CAN2_FDC_BCM_Acc5Sta_Sta : Outport
  wires:
  Data Type Conversion/1 -> CAN2_FDC_BCM_Acc5Sta_Sta/1
  FDCBCMAcc5StaSta/1 -> Data Type Conversion/1

== system halout/HAL_OUT/CAN2/FD2_CE200_1_0x435/FDCBCMAmbBrightStaSta ==
  FDCBCMAmbBrightStaSta : Inport
  Data Type Conversion : DataTypeConversion  OutDataTypeStr=uint8  RndMeth=Round
  CAN2_FDC_BCM_AmbBrightSta_Sta : Outport
  wires:
  Data Type Conversion/1 -> CAN2_FDC_BCM_AmbBrightSta_Sta/1
  FDCBCMAmbBrightStaSta/1 -> Data Type Conversion/1

== system halout/HAL_OUT/CAN2/FD2_CE200_1_0x435/FDCBCMAmbColorStaSta ==
  FDCBCMAmbColorStaSta : Inport
  Data Type Conversion : DataTypeConversion  OutDataTypeStr=uint8  RndMeth=Round
  CAN2_FDC_BCM_AmbColorSta_Sta : Outport
  wires:
  Data Type Conversion/1 -> CAN2_FDC_BCM_AmbColorSta_Sta/1
  FDCBCMAmbColorStaSta/1 -> Data Type Conversion/1

== system halout/HAL_OUT/CAN2/FD2_CE200_1_0x435/FDCBCMAmbDimENSta ==
  FDCBCMAmbDimENSta : Inport
  Data Type Conversion : DataTypeConversion  OutDataTypeStr=uint8  RndMeth=Round
  CAN2_FDC_BCM_AmbDimEN_Sta : Outport
  wires:
  Data Type Conversion/1 -> CAN2_FDC_BCM_AmbDimEN_Sta/1
  FDCBCMAmbDimENSta/1 -> Data Type Conversion/1

== system halout/HAL_OUT/CAN2/FD2_CE200_1_0x435/FDCBCMAmbFunENSta ==
  FDCBCMAmbFunENSta : Inport
  Data Type Conversion : DataTypeConversion  OutDataTypeStr=uint8  RndMeth=Round
  CAN2_FDC_BCM_AmbFunEN_Sta : Outport
  wires:
  Data Type Conversion/1 -> CAN2_FDC_BCM_AmbFunEN_Sta/1
  FDCBCMAmbFunENSta/1 -> Data Type Conversion/1

== system halout/HAL_OUT/CAN2/FD2_CE200_1_0x435/FDCBCMAmbLinkDriStaSta ==
  FDCBCMAmbLinkDriStaSta : Inport
  Data Type Conversion : DataTypeConversion  OutDataTypeStr=uint8  RndMeth=Round
  CAN2_FDC_BCM_AmbLinkDriSta_Sta : Outport
  wires:
  Data Type Conversion/1 -> CAN2_FDC_BCM_AmbLinkDriSta_Sta/1
  FDCBCMAmbLinkDriStaSta/1 -> Data Type Conversion/1

== system halout/HAL_OUT/CAN2/FD2_CE200_1_0x435/FDCBCMAmbODAENSta ==
  FDCBCMAmbODAENSta : Inport
  Data Type Conversion : DataTypeConversion  OutDataTypeStr=uint8  RndMeth=Round
  CAN2_FDC_BCM_AmbODAEN_Sta : Outport
  wires:
  Data Type Conversion/1 -> CAN2_FDC_BCM_AmbODAEN_Sta/1
  FDCBCMAmbODAENSta/1 -> Data Type Conversion/1

== system halout/HAL_OUT/CAN2/FD2_CE200_1_0x435/FDCBCMAmbPwrWarnENSta ==
  FDCBCMAmbPwrWarnENSta : Inport
  Data Type Conversion : DataTypeConversion  OutDataTypeStr=uint8  RndMeth=Round
  CAN2_FDC_BCM_AmbPwrWarnEN_Sta : Outport
  wires:
  Data Type Conversion/1 -> CAN2_FDC_BCM_AmbPwrWarnEN_Sta/1
  FDCBCMAmbPwrWarnENSta/1 -> Data Type Conversion/1

== system halout/HAL_OUT/CAN2/FD2_CE200_1_0x435/FDCBCMAmbWelENSta ==
  FDCBCMAmbWelENSta : Inport
  Data Type Conversion : DataTypeConversion  OutDataTypeStr=uint8  RndMeth=Round
  CAN2_FDC_BCM_AmbWelEN_Sta : Outport
  wires:
  Data Type Conversion/1 -> CAN2_FDC_BCM_AmbWelEN_Sta/1
  FDCBCMAmbWelENSta/1 -> Data Type Conversion/1

== system halout/HAL_OUT/CAN2/FD2_CE200_1_0x435/FDCBCMAutoLockSta ==
  FDCBCMAutoLockSta : Inport
  Data Type Conversion : DataTypeConversion  OutDataTypeStr=uint8  RndMeth=Round
  CAN2_FDC_BCM_AutoLock_Sta : Outport
  wires:
  Data Type Conversion/1 -> CAN2_FDC_BCM_AutoLock_Sta/1
  FDCBCMAutoLockSta/1 -> Data Type Conversion/1

== system halout/HAL_OUT/CAN2/FD2_CE200_1_0x435/FDCBCMAutoUnlockSta ==
  FDCBCMAutoUnlockSta : Inport
  Data Type Conversion : DataTypeConversion  OutDataTypeStr=uint8  RndMeth=Round
  CAN2_FDC_BCM_AutoUnlock_Sta : Outport
  wires:
  Data Type Conversion/1 -> CAN2_FDC_BCM_AutoUnlock_Sta/1
  FDCBCMAutoUnlockSta/1 -> Data Type Conversion/1

== system halout/HAL_OUT/CAN2/FD2_CE200_1_0x435/FDCBCMCLWinLockDrSta ==
  FDCBCMCLWinLockDrSta : Inport
  Data Type Conversion : DataTypeConversion  OutDataTypeStr=uint8  RndMeth=Round
  CAN2_FDC_BCM_CLWinLockDr_Sta : Outport
  wires:
  Data Type Conversion/1 -> CAN2_FDC_BCM_CLWinLockDr_Sta/1
  FDCBCMCLWinLockDrSta/1 -> Data Type Conversion/1

== system halout/HAL_OUT/CAN2/FD2_CE200_1_0x435/FDCBCMDSEATentryfsetSta ==
  FDCBCMDSEATentryfsetSta : Inport
  Data Type Conversion : DataTypeConversion  OutDataTypeStr=uint8  RndMeth=Round
  CAN2_FDC_BCM_DSEATentryfset_Sta : Outport
  wires:
  Data Type Conversion/1 -> CAN2_FDC_BCM_DSEATentryfset_Sta/1
  FDCBCMDSEATentryfsetSta/1 -> Data Type Conversion/1

== system halout/HAL_OUT/CAN2/FD2_CE200_1_0x435/FDCBCMFollowMeENFunSta ==
  FDCBCMFollowMeENFunSta : Inport
  Data Type Conversion : DataTypeConversion  OutDataTypeStr=uint8  RndMeth=Round
  CAN2_FDC_BCM_FollowMeENFun_Sta : Outport
  wires:
  Data Type Conversion/1 -> CAN2_FDC_BCM_FollowMeENFun_Sta/1
  FDCBCMFollowMeENFunSta/1 -> Data Type Conversion/1

== system halout/HAL_OUT/CAN2/FD2_CE200_1_0x435/FDCBCMKey10AccSta ==
  FDCBCMKey10AccSta : Inport
  Data Type Conversion : DataTypeConversion  OutDataTypeStr=uint8  RndMeth=Round
  CAN2_FDC_BCM_Key10Acc_Sta : Outport
  wires:
  Data Type Conversion/1 -> CAN2_FDC_BCM_Key10Acc_Sta/1
  FDCBCMKey10AccSta/1 -> Data Type Conversion/1

== system halout/HAL_OUT/CAN2/FD2_CE200_1_0x435/FDCBCMKey1AccSta ==
  FDCBCMKey1AccSta : Inport
  Data Type Conversion : DataTypeConversion  OutDataTypeStr=uint8  RndMeth=Round
  CAN2_FDC_BCM_Key1Acc_Sta : Outport
  wires:
  Data Type Conversion/1 -> CAN2_FDC_BCM_Key1Acc_Sta/1
  FDCBCMKey1AccSta/1 -> Data Type Conversion/1

== system halout/HAL_OUT/CAN2/FD2_CE200_1_0x435/FDCBCMKey2AccSta ==
  FDCBCMKey2AccSta : Inport
  Data Type Conversion : DataTypeConversion  OutDataTypeStr=uint8  RndMeth=Round
  CAN2_FDC_BCM_Key2Acc_Sta : Outport
  wires:
  Data Type Conversion/1 -> CAN2_FDC_BCM_Key2Acc_Sta/1
  FDCBCMKey2AccSta/1 -> Data Type Conversion/1

== system halout/HAL_OUT/CAN2/FD2_CE200_1_0x435/FDCBCMKey3AccSta ==
  FDCBCMKey3AccSta : Inport
  Data Type Conversion : DataTypeConversion  OutDataTypeStr=uint8  RndMeth=Round
  CAN2_FDC_BCM_Key3Acc_Sta : Outport
  wires:
  Data Type Conversion/1 -> CAN2_FDC_BCM_Key3Acc_Sta/1
  FDCBCMKey3AccSta/1 -> Data Type Conversion/1

== system halout/HAL_OUT/CAN2/FD2_CE200_1_0x435/FDCBCMKey4AccSta ==
  FDCBCMKey4AccSta : Inport
  Data Type Conversion : DataTypeConversion  OutDataTypeStr=uint8  RndMeth=Round
  CAN2_FDC_BCM_Key4Acc_Sta : Outport
  wires:
  Data Type Conversion/1 -> CAN2_FDC_BCM_Key4Acc_Sta/1
  FDCBCMKey4AccSta/1 -> Data Type Conversion/1

== system halout/HAL_OUT/CAN2/FD2_CE200_1_0x435/FDCBCMKey5AccSta ==
  FDCBCMKey5AccSta : Inport
  Data Type Conversion : DataTypeConversion  OutDataTypeStr=uint8  RndMeth=Round
  CAN2_FDC_BCM_Key5Acc_Sta : Outport
  wires:
  Data Type Conversion/1 -> CAN2_FDC_BCM_Key5Acc_Sta/1
  FDCBCMKey5AccSta/1 -> Data Type Conversion/1

== system halout/HAL_OUT/CAN2/FD2_CE200_1_0x435/FDCBCMKey6AccSta ==
  FDCBCMKey6AccSta : Inport
  Data Type Conversion : DataTypeConversion  OutDataTypeStr=uint8  RndMeth=Round
  CAN2_FDC_BCM_Key6Acc_Sta : Outport
  wires:
  Data Type Conversion/1 -> CAN2_FDC_BCM_Key6Acc_Sta/1
  FDCBCMKey6AccSta/1 -> Data Type Conversion/1

== system halout/HAL_OUT/CAN2/FD2_CE200_1_0x435/FDCBCMKey7AccSta ==
  FDCBCMKey7AccSta : Inport
  Data Type Conversion : DataTypeConversion  OutDataTypeStr=uint8  RndMeth=Round
  CAN2_FDC_BCM_Key7Acc_Sta : Outport
  wires:
  Data Type Conversion/1 -> CAN2_FDC_BCM_Key7Acc_Sta/1
  FDCBCMKey7AccSta/1 -> Data Type Conversion/1

== system halout/HAL_OUT/CAN2/FD2_CE200_1_0x435/FDCBCMKey8AccSta ==
  FDCBCMKey8AccSta : Inport
  Data Type Conversion : DataTypeConversion  OutDataTypeStr=uint8  RndMeth=Round
  CAN2_FDC_BCM_Key8Acc_Sta : Outport
  wires:
  Data Type Conversion/1 -> CAN2_FDC_BCM_Key8Acc_Sta/1
  FDCBCMKey8AccSta/1 -> Data Type Conversion/1

== system halout/HAL_OUT/CAN2/FD2_CE200_1_0x435/FDCBCMKey9AccSta ==
  FDCBCMKey9AccSta : Inport
  Data Type Conversion : DataTypeConversion  OutDataTypeStr=uint8  RndMeth=Round
  CAN2_FDC_BCM_Key9Acc_Sta : Outport
  wires:
  Data Type Conversion/1 -> CAN2_FDC_BCM_Key9Acc_Sta/1
  FDCBCMKey9AccSta/1 -> Data Type Conversion/1

== system halout/HAL_OUT/CAN2/FD2_CE200_1_0x435/FDCBCMLockAlarmCmd ==
  FDCBCMLockAlarmCmd : Inport
  Data Type Conversion : DataTypeConversion  OutDataTypeStr=uint8  RndMeth=Round
  CAN2_FDC_BCM_LockAlarm_Cmd : Outport
  wires:
  Data Type Conversion/1 -> CAN2_FDC_BCM_LockAlarm_Cmd/1
  FDCBCMLockAlarmCmd/1 -> Data Type Conversion/1

== system halout/HAL_OUT/CAN2/FD2_CE200_1_0x435/FDCBCMPTGOpenHeightSta ==
  FDCBCMPTGOpenHeightSta : Inport
  Data Type Conversion : DataTypeConversion  OutDataTypeStr=uint8  RndMeth=Round
  CAN2_FDC_BCM_PTGOpenHeight_Sta : Outport
  wires:
  Data Type Conversion/1 -> CAN2_FDC_BCM_PTGOpenHeight_Sta/1
  FDCBCMPTGOpenHeightSta/1 -> Data Type Conversion/1

== system halout/HAL_OUT/CAN2/FD2_CE200_1_0x435/FDCBCMRmLpModeENFunSta ==
  FDCBCMRmLpModeENFunSta : Inport
  Data Type Conversion : DataTypeConversion  OutDataTypeStr=uint8  RndMeth=Round
  CAN2_FDC_BCM_RmLpModeENFun_Sta : Outport
  wires:
  Data Type Conversion/1 -> CAN2_FDC_BCM_RmLpModeENFun_Sta/1
  FDCBCMRmLpModeENFunSta/1 -> Data Type Conversion/1

== system halout/HAL_OUT/CAN2/FD2_CE200_1_0x435/FDCBCMTurnSwTSetStaSta ==
  FDCBCMTurnSwTSetStaSta : Inport
  Data Type Conversion : DataTypeConversion  OutDataTypeStr=uint8  RndMeth=Round
  CAN2_FDC_BCM_TurnSwTSetSta_Sta : Outport
  wires:
  Data Type Conversion/1 -> CAN2_FDC_BCM_TurnSwTSetSta_Sta/1
  FDCBCMTurnSwTSetStaSta/1 -> Data Type Conversion/1

== system halout/HAL_OUT/CAN2/FD2_CE200_1_0x435/FDCBCMUserNowSta ==
  FDCBCMUserNowSta : Inport
  Data Type Conversion : DataTypeConversion  OutDataTypeStr=uint8  RndMeth=Round
  CAN2_FDC_BCM_UserNow_Sta : Outport
  wires:
  Data Type Conversion/1 -> CAN2_FDC_BCM_UserNow_Sta/1
  FDCBCMUserNowSta/1 -> Data Type Conversion/1

== system halout/HAL_OUT/CAN2/FD2_CE200_1_0x435/FDCBCMWalkInUnLkEnFunSta ==
  FDCBCMWalkInUnLkEnFunSta : Inport
  Data Type Conversion : DataTypeConversion  OutDataTypeStr=uint8  RndMeth=Round
  CAN2_FDC_BCM_WalkInUnLkEnFun_Sta : Outport
  wires:
  Data Type Conversion/1 -> CAN2_FDC_BCM_WalkInUnLkEnFun_Sta/1
  FDCBCMWalkInUnLkEnFunSta/1 -> Data Type Conversion/1

== system halout/HAL_OUT/CAN2/FD2_CE200_1_0x435/FDCBCMWalkOutLkEnFunSta ==
  FDCBCMWalkOutLkEnFunSta : Inport
  Data Type Conversion : DataTypeConversion  OutDataTypeStr=uint8  RndMeth=Round
  CAN2_FDC_BCM_WalkOutLkEnFun_Sta : Outport
  wires:
  Data Type Conversion/1 -> CAN2_FDC_BCM_WalkOutLkEnFun_Sta/1
  FDCBCMWalkOutLkEnFunSta/1 -> Data Type Conversion/1

== system halout/HAL_OUT/CAN2/FD2_CE200_1_0x435/FDCDKCDkeyShowIVISta ==
  FDCDKCDkeyShowIVISta : Inport
  Data Type Conversion : DataTypeConversion  OutDataTypeStr=uint8  RndMeth=Round
  CAN2_FDC_DKC_DkeyShowIVI_Sta : Outport
  wires:
  Data Type Conversion/1 -> CAN2_FDC_DKC_DkeyShowIVI_Sta/1
  FDCDKCDkeyShowIVISta/1 -> Data Type Conversion/1

== system halout/HAL_OUT/CAN2/FD2_CE200_1_0x435/FDCDKCKeyMissSta ==
  FDCDKCKeyMissSta : Inport
  Data Type Conversion : DataTypeConversion  OutDataTypeStr=uint8  RndMeth=Round
  CAN2_FDC_DKC_KeyMiss_Sta : Outport
  wires:
  Data Type Conversion/1 -> CAN2_FDC_DKC_KeyMiss_Sta/1
  FDCDKCKeyMissSta/1 -> Data Type Conversion/1

== system halout/HAL_OUT/CAN2/FD2_CE200_1_0x435/FDCDKCKeyNumSta ==
  FDCDKCKeyNumSta : Inport
  Data Type Conversion : DataTypeConversion  OutDataTypeStr=uint8  RndMeth=Round
  CAN2_FDC_DKC_KeyNum_Sta : Outport
  wires:
  Data Type Conversion/1 -> CAN2_FDC_DKC_KeyNum_Sta/1
  FDCDKCKeyNumSta/1 -> Data Type Conversion/1

== system halout/HAL_OUT/CAN2/FD2_CE200_1_0x435/FDCDKCKeyTypeSta ==
  FDCDKCKeyTypeSta : Inport
  Data Type Conversion : DataTypeConversion  OutDataTypeStr=uint8  RndMeth=Round
  CAN2_FDC_DKC_KeyType_Sta : Outport
  wires:
  Data Type Conversion/1 -> CAN2_FDC_DKC_KeyType_Sta/1
  FDCDKCKeyTypeSta/1 -> Data Type Conversion/1

== system halout/HAL_OUT/CAN2/FD2_CE200_1_0x435/FDCDKCUIDLowPowerSta ==
  FDCDKCUIDLowPowerSta : Inport
  Data Type Conversion : DataTypeConversion  OutDataTypeStr=uint8  RndMeth=Round
  CAN2_FDC_DKC_UIDLowPower_Sta : Outport
  wires:
  Data Type Conversion/1 -> CAN2_FDC_DKC_UIDLowPower_Sta/1
  FDCDKCUIDLowPowerSta/1 -> Data Type Conversion/1

== system halout/HAL_OUT/CAN2/FD2_CE200_1_0x435/FDCFGSAirIntSta ==
  FDCFGSAirIntSta : Inport
  Data Type Conversion : DataTypeConversion  OutDataTypeStr=uint8  RndMeth=Round
  CAN2_FDC_FGS_AirInt_Sta : Outport
  wires:
  Data Type Conversion/1 -> CAN2_FDC_FGS_AirInt_Sta/1
  FDCFGSAirIntSta/1 -> Data Type Conversion/1

== system halout/HAL_OUT/CAN2/FD2_CE200_1_0x435/FDCFGSFGSChSta ==
  FDCFGSFGSChSta : Inport
  Data Type Conversion : DataTypeConversion  OutDataTypeStr=uint8  RndMeth=Round
  CAN2_FDC_FGS_FGSCh_Sta : Outport
  wires:
  Data Type Conversion/1 -> CAN2_FDC_FGS_FGSCh_Sta/1
  FDCFGSFGSChSta/1 -> Data Type Conversion/1

== system halout/HAL_OUT/CAN2/FD2_CE200_1_0x435/FDCFGSIONSWSta ==
  FDCFGSIONSWSta : Inport
  Data Type Conversion : DataTypeConversion  OutDataTypeStr=uint8  RndMeth=Round
  CAN2_FDC_FGS_IONSW_Sta : Outport
  wires:
  Data Type Conversion/1 -> CAN2_FDC_FGS_IONSW_Sta/1
  FDCFGSIONSWSta/1 -> Data Type Conversion/1

== system halout/HAL_OUT/CAN2/FD2_CE200_1_0x435/FDCSPTGSPTGENFunSta ==
  FDCSPTGSPTGENFunSta : Inport
  Data Type Conversion : DataTypeConversion  OutDataTypeStr=uint8  RndMeth=Round
  CAN2_FDC_SPTG_SPTGENFun_Sta : Outport
  wires:
  Data Type Conversion/1 -> CAN2_FDC_SPTG_SPTGENFun_Sta/1
  FDCSPTGSPTGENFunSta/1 -> Data Type Conversion/1
